simulink model "TwoWheelFuzzy"  (R2024b)
settings: Solver=VariableStepAuto  StartTime=0.0  StopTime=2.7  RelTol=1e-3
libraries: fuzblock x2
settings Model: Creator=Dr.Red  LastModifiedBy=Dr.Red

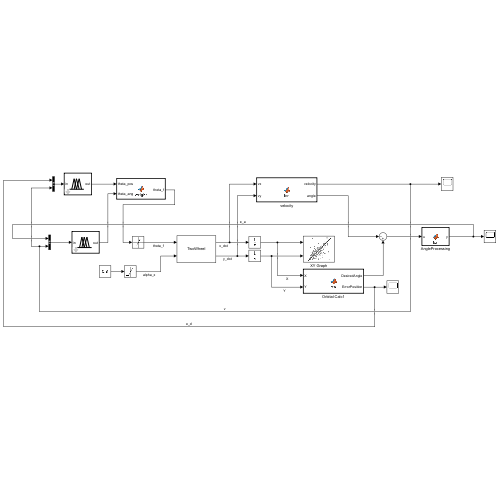
[thumbnail: Simulink's stored preview of the top-level diagram]
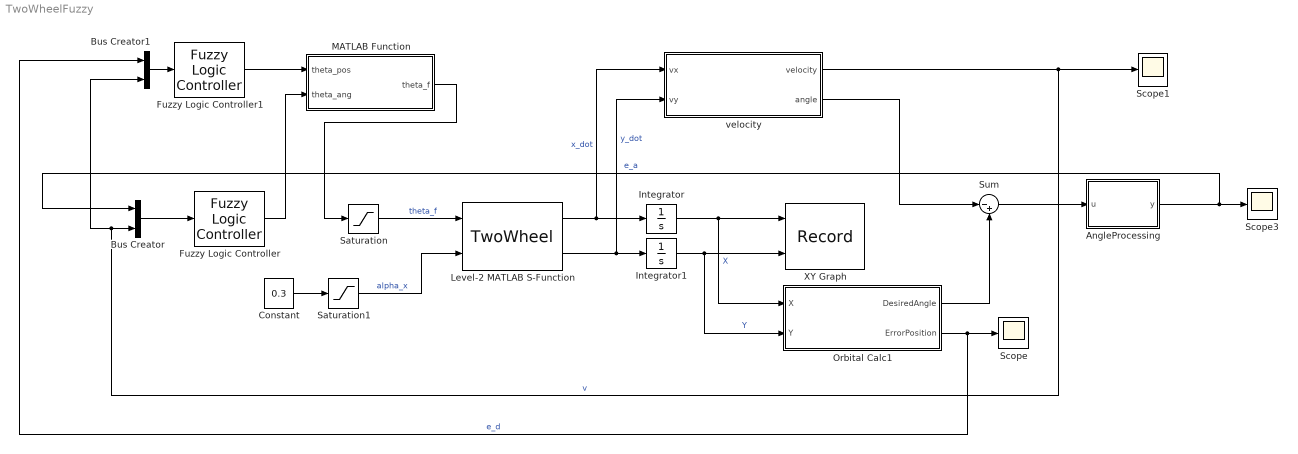
== system TwoWheelFuzzy ==
  AngleProcessing : MATLAB Function  TreatAsAtomicUnit=on
  Bus Creator : BusCreator  Inputs=2
  Bus Creator1 : BusCreator  Inputs=2
  Constant : Constant  Value=0.3
  Fuzzy Logic Controller : fuzblock/Fuzzy Logic  Controller  FIS='Fuzzy.fis'  OutputSampleNumber=101  DataType=double  FuzzifiedInputs=off  RuleFiringStrengths=off  RuleOutputs=off  AggregatedOutputs=off  SimulateUsing=Interpreted execution  OutOfRangeInputValueMessage=warning  NoRuleFiredMessage=warning  EmptyOutputFuzzySetMessage=warning
  Fuzzy Logic Controller1 : fuzblock/Fuzzy Logic  Controller  FIS='Fuzzy2.fis'  OutputSampleNumber=101  DataType=double  FuzzifiedInputs=off  RuleFiringStrengths=off  RuleOutputs=off  AggregatedOutputs=off  SimulateUsing=Interpreted execution  OutOfRangeInputValueMessage=warning  NoRuleFiredMessage=warning  EmptyOutputFuzzySetMessage=warning
  Integrator : Integrator
  Integrator1 : Integrator
  Level-2 MATLAB S-Function : M-S-Function  FunctionName=TwoWheel  Parameters=8,0,0,0
  MATLAB Function : MATLAB Function  TreatAsAtomicUnit=on
  Orbital Calc1 : MATLAB Function  TreatAsAtomicUnit=on
  Saturation : Saturate  UpperLimit=0.3  LowerLimit=-0.3
  Saturation1 : Saturate  UpperLimit=1.5  LowerLimit=-1.5
  Scope : Scope
  Scope1 : Scope
  Scope3 : Scope
  Sum : Sum  Inputs=|-+
  XY Graph : Record  FileSettingsInternal="{\"entries\":[{\"content\":{\"excelSettings\":{\"content\":{},\"type\":\"Streamout.ExcelSettings\"}},\"type\":\"Streamout.FileSettingStorage\",\"uuid\":\"\"}],\"packageUris\":[\"http:\\/\\/schema.mathworks.com\\/mf0\\/streamout_blocks\\/R2020a\"],\"version\":\"1.0\"}"  Layout=[1 1]  SignalsInternal="{\"entries\":[{\"content\":{\"signals\":[{\"content\":{\"blockPath\":[],\"dimensions\":[1],\"domain\":\"\",\"lineColor\":\"#a2142f\",\"plots\":[ 1 ],\"port\":1,\"sid\":[\"\"],\"signalID\":1,\"signalName\":\"X\"},\"type\":\"RecordBlkView.Signal\",\"uuid\":\"\"},{\"content\":{\"blockPath\":[],\"dimensions\":[1],\"domain\":\"\",\"lineColor\":\"#139fff\",\"plots\":[ 1 ],\"port\":2,\"sid\":[\"\"],\"signalID\":2,\"signalName\":\"Y\"},\"type\":\"RecordBlkView.Signal\",\"uuid\":\"\"}]},\"type\":\"RecordBlkView.InputSignals\",\"uuid\":\"\"}],\"packageUris\":[\"http:\\/\\/schema.mathworks.com\\/mf0\\/streamout_blocks\\/R2020a\"],\"version\":\"1.0\"}"  VisualizationBindings="{\"xyplotplugin\":{\"info\":[{\"series\":[{\"bindingParametersList\":[{\"parameter\":\"X-Axis\",\"signalID\":1,\"signalName\":\"X\"},{\"parameter\":\"Y-Axis\",\"signalID\":2,\"signalName\":\"Y\"}],\"seriesID\":0}],\"subplotID\":1}]}}"  CompatibilityTag=XY
  velocity : MATLAB Function  TreatAsAtomicUnit=on
  wires:
  velocity/2(angle) -> Sum/1
  velocity/1(velocity) -> Bus Creator1/2, Bus Creator/2, Scope1/1  "v"
  Orbital Calc1/1(DesiredAngle) -> Sum/2
  Saturation/1 -> Level-2 MATLAB S-Function/1  "theta_f"
  Integrator/1 -> XY Graph/1, Orbital Calc1/1(X)  "X"
  Level-2 MATLAB S-Function/1 -> velocity/1(vx), Integrator/1  "x_dot"
  Integrator1/1 -> Orbital Calc1/2(Y), XY Graph/2  "Y"
  Sum/1 -> AngleProcessing/1(u)
  Level-2 MATLAB S-Function/2 -> velocity/2(vy), Integrator1/1  "y_dot"
  Bus Creator/1 -> Fuzzy Logic Controller/1
  Bus Creator1/1 -> Fuzzy Logic Controller1/1
  Fuzzy Logic Controller1/1 -> MATLAB Function/1(theta_pos)
  Fuzzy Logic Controller/1 -> MATLAB Function/2(theta_ang)
  MATLAB Function/1(theta_f) -> Saturation/1
  AngleProcessing/1(y) -> Bus Creator/1, Scope3/1  "e_a"
  Saturation1/1 -> Level-2 MATLAB S-Function/2  "alpha_x"
  Constant/1 -> Saturation1/1
  Orbital Calc1/2(ErrorPosition) -> Bus Creator1/1, Scope/1  "e_d"

== matlab function TwoWheelFuzzy/MATLAB Function ==
  data: theta_pos input; theta_ang input; theta_f output
function theta_f = weight(theta_pos,theta_ang)
    w = 0.4;
    theta_pos = theta_pos + 0.393;

theta_f = theta_ang*w+theta_pos*(1-w);

== matlab function TwoWheelFuzzy/AngleProcessing ==
  data: u input; y output
function y = fcn(u)

y = mod(u + pi, 2*pi) - pi;

== matlab function TwoWheelFuzzy/Orbital Calc1 ==
  data: DesiredAngle output; X input; ErrorPosition output; Y input
function [DesiredAngle,ErrorPosition] = fcn(X,Y)
    
    RoundPosition = [0,15];

    Radius = 15;

ErrorPosition = - Radius + power((RoundPosition(1)-X)^2+(RoundPosition(2)-Y)^2,0.5);

DesiredAngle = atan2(X-RoundPosition(1),RoundPosition(2)-Y);

== matlab function TwoWheelFuzzy/velocity ==
  data: vx input; velocity output; vy input; angle output
function [velocity,angle] = fcn(vx,vy)
    

velocity = power(vx^2+vy^2,0.5);

angle = atan2(vy,vx);
